simulink model "arduino_imu_pitch_roll"  (R2022a)
settings: Solver=FixedStepAuto  StartTime=0.0  StopTime=inf  RelTol=1e-3  EnableMultiTasking=on
settings Model: ExtModeTrigDuration=2  Creator=The MathWorks, Inc.  LastModifiedBy=cwpan
settings SolverCC: AlgebraicLoopSolver=TrustRegion
settings DataIOCC: ReturnWorkspaceOutputs=off
settings OptimizationCC: EnhancedBackFolding=on  PassReuseOutputArgsThreshold=0  MaxStackSize=64  OptimizeBlockOrder=speed  DifferentSizesBufferReuse=on  OptimizationCustomize=off
settings DebuggingCC: ParameterTunabilityLossMsg=error  UnconnectedInputMsg=warning  UnconnectedOutputMsg=warning  UnconnectedLineMsg=warning  SFMachineParentedDataDiag=warning
settings HardwareCC: ProdBitPerInt=16  ProdBitPerPointer=16  ProdBitPerSizeT=16  ProdBitPerPtrDiffT=16  ProdLargestAtomicFloat=None  ProdWordSize=8  ProdHWDeviceType=Atmel->AVR  UseEmbeddedCoderFeatures=off  UseSimulinkCoderFeatures=off
settings SFSimCC: MATLABDynamicMemAlloc=off
settings RTWCC: SystemTargetFile=ert.tlc  HardwareBoard=Arduino Uno  TemplateMakefile=ert_default_tmf  Toolchain=Arduino AVR  BuildConfiguration=Faster Runs  DLArmComputeVersion=19.05
settings CodeAppCC: ForceParamTrailComments=on  OperatorAnnotations=on
settings ERTTargetCC: ERTCustomFileBanners=off  SupportContinuousTime=on  SupportNonInlinedSFcns=on  RemoveResetFunc=off  SupportVariableSizeSignals=on  ModelStepFunctionPrototypeControlCompliant=off  ExtModeTransport=3  ExtModeStaticAlloc=on  ExtModeStaticAllocSize=250  ExtModeMexFile=ext_xcp  ExtModeIntrfLevel=Level2 - Open

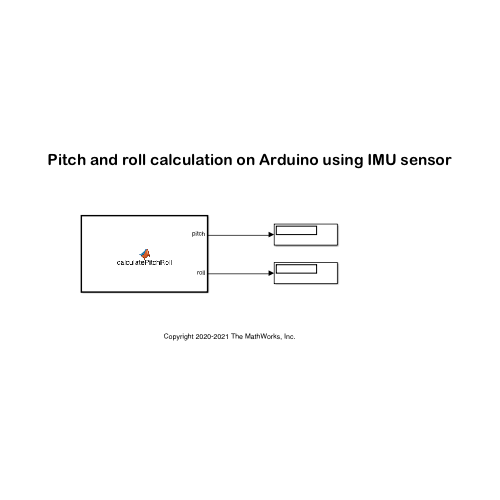
[thumbnail: Simulink's stored preview of the top-level diagram]
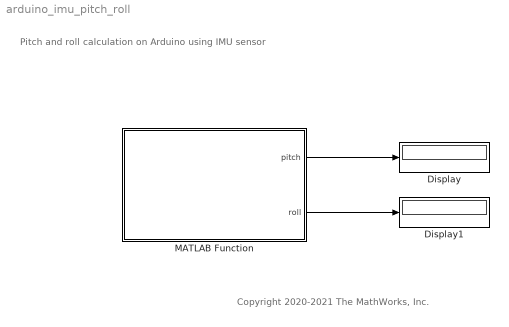
== system arduino_imu_pitch_roll ==
  note: Copyright 2020-2021 The MathWorks, Inc.
  note: Pitch and roll calculation on Arduino using IMU sensor
  Display : Display
  Display1 : Display
  MATLAB Function : MATLAB Function  TreatAsAtomicUnit=on  SystemSampleTime=1/100
  wires:
  MATLAB Function/1(pitch) -> Display/1
  MATLAB Function/2(roll) -> Display1/1

== matlab function arduino_imu_pitch_roll/MATLAB Function ==
  data: pitch output; roll output
function [pitch, roll] = calculatePitchRoll()

% This function reads acceleration and angular velocity from an IMU sensor
% and calculates its orientation by finding out pitch and roll. In this
% application MPU9250 sensor is used. However, it could be replaced with
% any other IMU sensor as well.

persistent arduinoObj imuObj
persistent prevTimestamp
persistent pitchAngle rollAngle
persistent pitchAccelOffset rollAccelOffset pitchGyroOffset rollGyroOffset

% Output
roll = 0;
pitch = 0;

if isempty(arduinoObj)
    arduinoObj = arduino();
end
if isempty(imuObj)
    imuObj = lsm9ds1(arduinoObj);
end

% x -> longitudinal axis or N axis or roll axis
% y -> transverse axis or E axis or pitch axis
% z -> vertical axis or  D axis or yaw axis
if isempty(pitchAccelOffset)
pitchAccelOffset = 0;
pitchGyroOffset = 0;
rollAccelOffset = 0;
rollGyroOffset = 0;
prevTimestamp = 0;

% Calculate the average offset error produced by accelerometer and gyroscope.
count = 100;
for i = 1:count
    if i == count
        [accel, gyro, ~, timestamp] = read(imuObj);
        prevTimestamp = timestamp;
    else
        [accel, gyro] = read(imuObj);
    end
    pitchAccelOffset = pitchAccelOffset + atan2(accel(1), sqrt(accel(2)*accel(2) + accel(3)*accel(3)));
    rollAccelOffset = rollAccelOffset + atan2(-accel(2), sqrt(accel(1)*accel(1) + accel(3)*accel(3)));
    pitchGyroOffset = pitchGyroOffset + gyro(2);
    rollGyroOffset = rollGyroOffset + gyro(1);
end

pitchAccelOffset = pitchAccelOffset/count;
rollAccelOffset = rollAccelOffset/count;
pitchGyroOffset = pitchGyroOffset/count;
rollGyroOffset = rollGyroOffset/count;
end

if isempty(pitchAngle)
    pitchAngle = 0;
end

if isempty(rollAngle)
    rollAngle = 0;
end

% Using complementary filter to fuse accelerometer and gyroscope data.
% Filter coefficient should be tuned to improve result
filterCoeff = 0.98;

[accel, gyro, ~, timestamp] = read(imuObj);
% Calculate pitch and roll from acceleration values and remove offset
accelPitchAngle = atan2(accel(1), sqrt(accel(2)*accel(2) + accel(3)*accel(3))) - pitchAccelOffset;
accelRollAngle = atan2(-accel(2), sqrt(accel(1)*accel(1) + accel(3)*accel(3))) - rollAccelOffset;
% Subtract the offset values calculated at the beginning
gyro(1) = gyro(1) - rollGyroOffset;
gyro(2) = gyro(2) - pitchGyroOffset;
gyroPitchAngleDiff = gyro(2)*(timestamp - prevTimestamp);
gyroRollAngleDiff = gyro(1)*(timestamp - prevTimestamp);
prevTimestamp = timestamp;

% Use complementary filter to fuse accelerometer and gyroscope data
pitchAngle = filterCoeff*(pitchAngle + gyroPitchAngleDiff) + (1 - filterCoeff)*accelPitchAngle;
rollAngle = filterCoeff*(rollAngle + gyroRollAngleDiff) + (1 - filterCoeff)*accelRollAngle;

% sensor object returns angular velocity in radians/s. Converting pitch and
% roll angles into degree
pitch = pitchAngle*180/pi;
roll = rollAngle*180/pi;
